simulink model "pruebacontroladorclase"  (Simulink 7.9)
settings: Solver=ode45  StartTime=0.0  StopTime=100  RelTol=1e-3
settings Model: Creator=Miguel Faggioni  LastModifiedBy=Miguel Faggioni

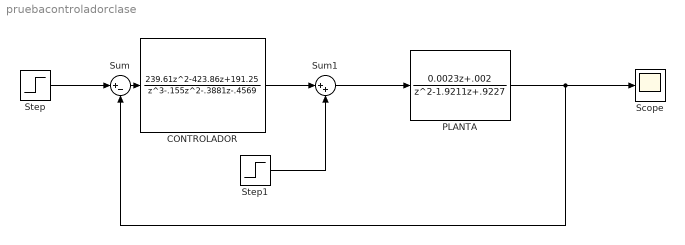
== system pruebacontroladorclase ==
  CONTROLADOR : DiscreteTransferFcn  Numerator=[239.61 -423.86 191.25]  Denominator=[1 -.155 -.3881 -.4569]
  PLANTA : DiscreteTransferFcn  Numerator=[0.0023 .002]  Denominator=[1 -1.9211 .9227]
  Scope : Scope
  Step : Step  Time=0  SampleTime=.5
  Step1 : Step  Time=50  SampleTime=.5
  Sum : Sum  Inputs=|+-
  Sum1 : Sum  Inputs=|++
  wires:
  PLANTA/1 -> Scope/1, Sum/2
  Step/1 -> Sum/1
  Sum/1 -> CONTROLADOR/1
  Step1/1 -> Sum1/2
  CONTROLADOR/1 -> Sum1/1
  Sum1/1 -> PLANTA/1
